simulink model "closedloop_pid"  (R2020a)
settings: Solver=VariableStepAuto  StartTime=0.0  StopTime=60  FixedStep=1e-4  RelTol=1e-6  EnableMultiTasking=on
libraries: cstblocks x2, simulink x1
settings Model: Creator=henrik  LastModifiedBy=henrik
settings DataIOCC: LimitDataPoints=on  SaveFormat=Array  SignalLoggingSaveFormat=ModelDataLogs  ReturnWorkspaceOutputs=off  SignalLoggingName=sigsOut
settings OptimizationCC: ExpressionDepthLimit=2147483647  InitFltsAndDblsToZero=on  LifeSpan=inf
settings DebuggingCC: SaveWithParameterizedLinksMsg=none  UnderspecifiedInitializationDetection=Classic  MergeDetectMultiDrivingBlocksExec=none  SignalResolutionControl=TryResolveAllWithWarning  MultiTaskDSMMsg=warning  MultiTaskCondExecSysMsg=none  FcnCallInpInsideContextMsg=warning  StateNameClashWarn=warning  SFUnexpectedBacktrackingDiag=warning  SFNoUnconditionalDefaultTransitionDiag=warning  SFExecutionAtInitializationDiag=none  ArithmeticOperatorsInVariantConditions=warning
settings HardwareCC: ProdBitPerPointer=32  ProdBitPerSizeT=32  ProdBitPerPtrDiffT=32  ProdLargestAtomicFloat=None  ProdIntDivRoundTo=Undefined  ProdEndianess=Unspecified  ProdWordSize=32  ProdHWDeviceType=32-bit Generic  TargetUnknown=on
settings ModelReferenceCC: PropagateSignalLabelsOutOfModel=off
settings SFSimCC: SimUseLocalCustomCode=off  CustomCodeUndefinedFunction=UseInterfaceOnly
settings RTWCC: RTWUseLocalCustomCode=off
settings CodeAppCC: StateflowObjectComments=on
settings GRTTargetCC: TargetFcnLib=ansi_tfl_tmw.mat  TargetLangStandard=C89/C90 (ANSI)  ModelReferenceCompliant=off  CombineOutputUpdateFcns=off  MatFileLogging=off  GRTInterface=on
settings ConfigComp: CovMetricSettings=dw  CovSaveCumulativeToWorkspaceVar=on  CovSaveSingleToWorkspaceVar=on  CovExternalEMLEnable=off  CovSFcnEnable=off

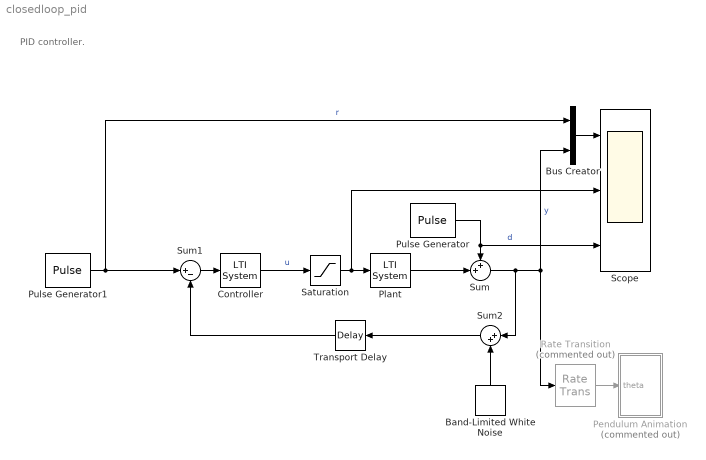
== system closedloop_pid ==
  note: PID controller.
  Band-Limited White Noise : simulink/Sources/Band-Limited White Noise  Cov=[0.000001]*0  Ts=0.01  seed=[23341]
  Bus Creator : BusCreator  Inputs=2
  Controller : cstblocks/LTI System  sys=C1  IC=[]
  Pendulum Animation : Subsystem  Commented=on
  Plant : cstblocks/LTI System  sys=Po  IC=[]
  Pulse Generator : DiscretePulseGenerator  PulseType=Time based  Amplitude=0.5  Period=60  PulseWidth=50  PhaseDelay=30
  Pulse Generator1 : DiscretePulseGenerator  PulseType=Time based  Amplitude=0.3  Period=1000  PulseWidth=50
  Rate Transition : RateTransition  Commented=on  OutPortSampleTime=0.05
  Saturation : Saturate  UpperLimit=inf  LowerLimit=-inf
  Scope : Scope  NumInputPorts=3
  Sum : Sum  Inputs=++|  SaturateOnIntegerOverflow=on
  Sum1 : Sum  Inputs=|+-  SaturateOnIntegerOverflow=on
  Sum2 : Sum  Inputs=|++  SaturateOnIntegerOverflow=on
  Transport Delay : TransportDelay  DelayTime=1e-2*0
  wires:
  Controller/1 -> Saturation/1  "u"
  Pulse Generator/1 -> Sum/1, Scope/3  "d"
  Pulse Generator1/1 -> Bus Creator/1, Sum1/1  "r"
  Bus Creator/1 -> Scope/1
  Sum/1 -> Rate Transition/1, Bus Creator/2, Sum2/1  "y"
  Sum1/1 -> Controller/1
  Sum2/1 -> Transport Delay/1
  Band-Limited White Noise/1 -> Sum2/2
  Plant/1 -> Sum/2
  Rate Transition/1 -> Pendulum Animation/1(theta)
  Transport Delay/1 -> Sum1/2
  Saturation/1 -> Scope/2, Plant/1

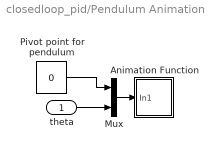
== system closedloop_pid/Pendulum Animation ==
  theta : Inport
  Animation Function : Subsystem  mask(Animation Block){ts=0.01}
      mask prompts: ts "Sample time:"
      mask Display: plot([.1,.9],[.9,.9],[.5,.2],[.9,.25],[.475,.475,.525,.525,.475],[.875,.925,.925,.875,.875])
  Mux : Mux  Inputs=2
  Pivot point for pendulum : Constant  Value=0
  wires:
  Mux/1 -> Animation Function/1(In1)
  Pivot point for pendulum/1 -> Mux/1
  theta/1 -> Mux/2

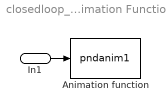
== system closedloop_pid/Pendulum Animation/Animation Function ==
  In1 : Inport
  Animation function : S-Function  FunctionName=pndanim1  Parameters=ts  SFunctionDeploymentMode=off  EnableBusSupport=off
      settings: DeleteFcn=if ~isempty(findobj('type','figure','name','simppend Animation'));close('simppend Animation'); end;
  wires:
  In1/1 -> Animation function/1
